simulink model "Kinematics"  (R2024b)
settings: Solver=VariableStepAuto  StartTime=0.0  StopTime=10.0  RelTol=1e-3
values from neighbouring files (symbols this model uses):
  q = [q_vect; q4]    [model.m]
undefined symbols (not defined in the file or in its folder): w
settings Model: Creator=sstef  LastModifiedBy=sstef

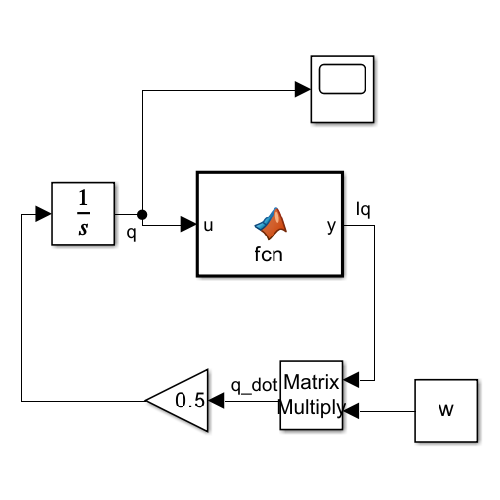
[thumbnail: Simulink's stored preview of the top-level diagram]
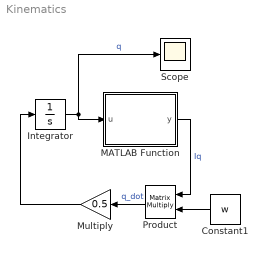
== system Kinematics ==
  Constant1 : Constant  Value=w
  Integrator : Integrator  InitialCondition=q
  MATLAB Function : MATLAB Function  TreatAsAtomicUnit=on
  Multiply : Gain  Gain=0.5
  Product : Product  Multiplication=Matrix(*)
  Scope : Scope
  wires:
  Integrator/1 -> Scope/1, MATLAB Function/1(u)  "q"
  Product/1 -> Multiply/1  "q_dot"
  MATLAB Function/1(y) -> Product/1  "Iq"
  Constant1/1 -> Product/2
  Multiply/1 -> Integrator/1

== matlab function Kinematics/MATLAB Function ==
  data: u input size=4 1; y output size=4 3
function y  = fcn(u)
q4=u(4);
q_vect=u(1:3);
qx=[0,  -q_vect(3)  q_vect(2);
    q_vect(3), 0,  -q_vect(1);
    -q_vect(2), q_vect(1), 0];

Iq=[eye(3)*q4+qx;
      -q_vect.'  ];
y = Iq;
